simulink model "Flyback"  (R2024b)
settings: Solver=ode4  StartTime=0.0  StopTime=2  FixedStep=1e-6  MaxStep=1e-4  RelTol=1e-3
values from neighbouring files (symbols this model uses):
  fs = 100e3    (= 100000)    [Tp_.m]
libraries: spsSeriesRLCBranchLib x2, spsControlledVoltageSourceLib x1, spsCurrentMeasurementLib x1, spsDiodeLib x1, spsIGBTDiodeLib x1, spsLinearTransformerLib x1, simulink x1, spsVariableResistorLib x1, spsVoltageMeasurementLib x1, spspowerguiLib x1
settings Model: Creator=ANIMESH SINHA  LastModifiedBy=asus
settings SolverCC: AlgebraicLoopSolver=TrustRegion
settings DataIOCC: ReturnWorkspaceOutputs=off
settings DebuggingCC: UnconnectedInputMsg=warning  UnconnectedOutputMsg=warning  UnconnectedLineMsg=warning  ArithmeticOperatorsInVariantConditions=warning
settings ModelReferenceCC: EnableRefExpFcnMdlSchedulingChecks=on
settings SFSimCC: SimUseLocalCustomCode=off  CustomCodeUndefinedFunction=UseInterfaceOnly
settings RTWCC: RTWUseLocalCustomCode=off  GPUComputeCapability=3.5
settings CodeAppCC: StateflowObjectComments=on
settings SimscapeCC: SimscapeNormalizeSystem=off

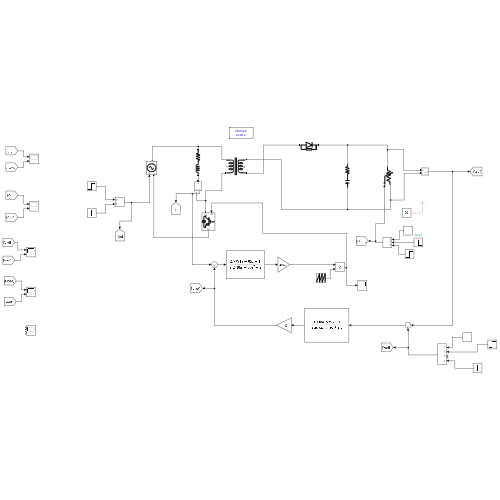
[thumbnail: Simulink's stored preview of the top-level diagram]
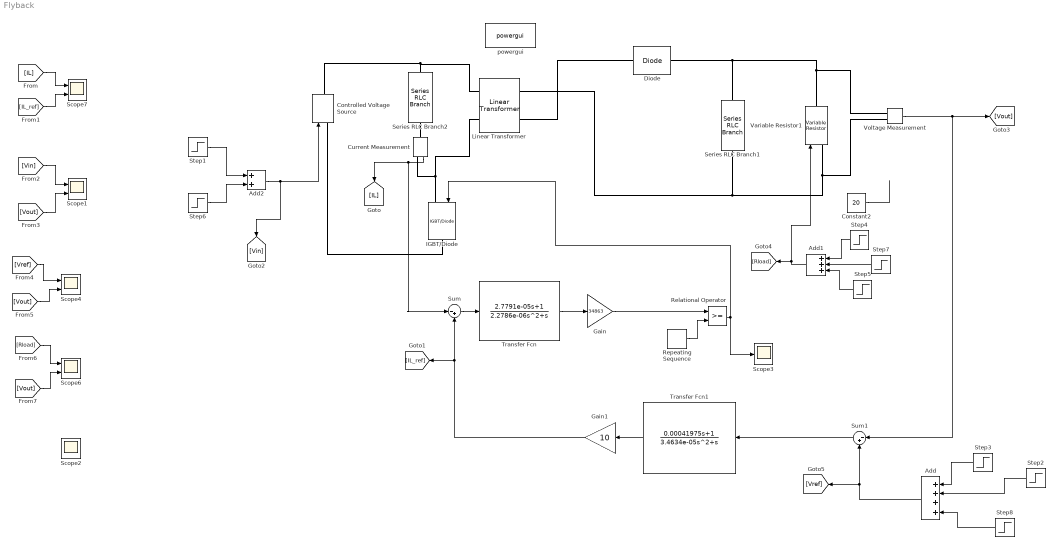
== system Flyback ==
  Add : Sum  Inputs=++++
  Add1 : Sum  Inputs=+++
  Add2 : Sum
  Constant2 : Constant  Value=20
  Controlled Voltage Source : spsControlledVoltageSourceLib/Controlled Voltage Source  Initialize=on  Source_Type=DC  Amplitude=0  Phase=0  Frequency=0  Measurements=None
  Current Measurement : spsCurrentMeasurementLib/Current Measurement  PhasorSimulation=off  OutputType=Complex  PSBequivalent=0
  Diode : spsDiodeLib/Diode  Ron=0.0001  Lon=0  Vf=0  IC=0  UseSnubber=0  Rs=500  Cs=inf  Measurements=off
  Gain : Gain  Gain=34863
  Gain1 : Gain  Gain=10
  IGBT/Diode : spsIGBTDiodeLib/IGBT//Diode  Ron=10e-3  Rs=1e5  Cs=inf  Measurements=off
  Linear Transformer : spsLinearTransformerLib/Linear Transformer  UNITS=SI  NominalPower=[100 100e3 ]  winding1=[12 0.2 0]  winding2=[4 0.1 0]  ThreeWindings=off  winding3=[3.15e+05 0.7938 7.5802e-07]  RmLm=[1e3 1e6]  Measurements=None  DataType=on
  Relational Operator : RelationalOperator  OutDataTypeStr=boolean  RndMeth=Simplest  InputSameDT=off
  Repeating Sequence : simulink/Sources/Repeating Sequence  rep_seq_t=[0 1/fs]  rep_seq_y=[0 1]
  Scope{1..2,4,6..7} (5 alike) : Scope  NumInputPorts=2
  Scope3 : Scope
  Series RLC Branch1 : spsSeriesRLCBranchLib/Series RLC Branch  LConnTagsString=__new0  RConnTagsString=__new0  BranchType=RC  Resistance=0.01  Inductance=1e-3  SetiL0=off  InitialCurrent=0  Capacitance=150e-6  Setx0=off  InitialVoltage=0  Measurements=None
  Series RLC Branch2 : spsSeriesRLCBranchLib/Series RLC Branch  LConnTagsString=__new0  RConnTagsString=__new0  BranchType=RL  Resistance=0.8785  Inductance=200e-6  SetiL0=off  InitialCurrent=0  Capacitance=1e-6  Setx0=off  InitialVoltage=0  Measurements=None
  Step1 : Step  Time=0.2  Before=12  After=16  SampleTime=0
  Step2 : Step  Time=0.8  After=4  SampleTime=0
  Step3 : Step  Time=0.5  Before=4  After=6  SampleTime=0
  Step4 : Step  Time=1.1  Before=20  After=18  SampleTime=0
  Step5 : Step  Time=1.4  After=+2  SampleTime=0
  Step6 : Step  Time=0.3  After=-10  SampleTime=0
  Step7 : Step  Time=1.2  After=-3  SampleTime=0
  Step8 : Step  After=-2  SampleTime=0
  Sum : Sum  Inputs=|-+
  Sum1 : Sum  Inputs=|-+
  Transfer Fcn : TransferFcn  Numerator=[2.7791e-05 1]  Denominator=[2.2786e-06 1 0 ]
  Transfer Fcn1 : TransferFcn  Numerator=[0.00041975 1]  Denominator=[3.4634e-05 1 0]
  Variable Resistor1 : spsVariableResistorLib/Variable Resistor  Rabsmin=1e-3
      settings: LibrarySourceBlock=sps_lib/Passives/Variable Resistor
  Voltage Measurement : spsVoltageMeasurementLib/Voltage Measurement  PhasorSimulation=off  OutputType=Complex  PSBequivalent=0
  powergui : spspowerguiLib/powergui  Priority=1  SimulationMode=Discrete  SampleTime=1e-6  frequency=60  Iterations=50  frequencyindice=0  Pbase=100e6  ErrMax=1e-4  UnitsV=kV  UnitsW=MW  buscounter=0  FunctionMessages=off  echomessages=off  EnableUseOfTLC=off  CurrentSourceSwitches=off  DisableSnubberDevices=off  DisableRonSwitches=off  DisableVfSwitches=off  DisplayEquations=off  AutomaticDiscreteSolvers=off  SolverType=Tustin/Backward Euler (TBE)  Interpol=off  ExternalGateDelay=off  methode=off  Ts=100  x0status=blocks  SPID=on  SwTol=0  HookPort=off  NonlinearTolerance=1e-4  nMaxIteration=100  ContinueOnMaxIteration=off  RestoreLinks=warning  ResistiveCurrentMeasurement=off  Frange=[0:2:500]  Ylog=off  Xlog=on  ShowGrid=off  save=off  variable=ZData  structure=0  ZoomFFT=off  StartTime=0.0  cycles=1  DisplayStyle=1  fundamental=60  FreqAxis=off  MaxFrequency=1000  frequencyindicesteady=1  RmsSteady=1  display=off
  wires:
  Sum/1 -> Transfer Fcn/1
  Transfer Fcn/1 -> Gain/1
  Repeating Sequence/1 -> Relational Operator/2
  Gain/1 -> Relational Operator/1
  Relational Operator/1 -> Scope3/1, IGBT/Diode/1
  Current Measurement/1 -> [IL], Sum/1
  Voltage Measurement/1 -> [Vout], Sum1/1
  Transfer Fcn1/1 -> Gain1/1
  Add/1 -> [Vref], Sum1/2
  Step3/1 -> Add/1
  Step4/1 -> Add1/1
  Add1/1 -> Variable Resistor1/1, [Rload]
  Add2/1 -> Controlled Voltage Source/1, [Vin]
  Step1/1 -> Add2/1
  Step6/1 -> Add2/2
  Step7/1 -> Add1/2
  [IL] -> Scope7/1
  [IL_ref] -> Scope7/2
  [Vin] -> Scope1/1
  [Vout] -> Scope1/2
  [Vout] -> Scope4/2
  [Vref] -> Scope4/1
  [Rload] -> Scope6/1
  [Vout] -> Scope6/2
  Sum1/1 -> Transfer Fcn1/1
  Gain1/1 -> [IL_ref], Sum/2
  Constant2/1 -> ?
  Step2/1 -> Add/2
  Step5/1 -> Add1/3
  Step8/1 -> Add/4
  connections:
  Linear Transformer/LConn1 -- Controlled Voltage Source/RConn1 -- Series RLC Branch2/LConn1
  Linear Transformer/LConn2 -- Current Measurement/RConn1 -- IGBT/Diode/LConn1
  IGBT/Diode/RConn1 -- Controlled Voltage Source/LConn1
  Linear Transformer/RConn1 -- Variable Resistor1/LConn1 -- Voltage Measurement/LConn2 -- Series RLC Branch1/RConn1
  Linear Transformer/RConn2 -- Diode/LConn1
  Diode/RConn1 -- Variable Resistor1/RConn1 -- Voltage Measurement/LConn1 -- Series RLC Branch1/LConn1
  Series RLC Branch2/RConn1 -- Current Measurement/LConn1
